simulink model "lqr_design_model"  (R2024a)
settings: Solver=ode45  StartTime=0.0  StopTime=2  FixedStep=0.002  RelTol=1e-3  EnableMultiTasking=on
values from neighbouring files (symbols this model uses):
  A = [0, 0, 1, 0 ... (first row only)    [Torsion_1D_ABCD_eqns_student.m]
  B = Kg * eta_g * kt * eta_m * B / Rm    [Torsion_1D_ABCD_eqns_student.m]
  C = [1, 0, 0, 0 ... (first row only)    [Torsion_1D_ABCD_eqns_student.m]    (also in pid_design.m = pid(Kp, Ki, Kd))
  K = db2mag(12.15)    [pid_design.m]    (also in setup_torsion.m = d_torsion_1d_lqr(A,B))
libraries: quarc_library x2
settings Model: ExtModeTrigDuration=10000  Creator=quarc_user  LastModifiedBy=quarc_user
settings SolverCC: AlgebraicLoopSolver=TrustRegion  PositivePriorityOrder=on
settings DataIOCC: ReturnWorkspaceOutputs=off
settings DebuggingCC: UnconnectedInputMsg=warning  UnconnectedOutputMsg=warning  UnconnectedLineMsg=warning  ArithmeticOperatorsInVariantConditions=warning
settings ModelReferenceCC: EnableRefExpFcnMdlSchedulingChecks=on
settings SFSimCC: SimUseLocalCustomCode=off  CustomCodeUndefinedFunction=UseInterfaceOnly
settings RTWCC: Description=QUARC Win64 Target Using Toolchain  SystemTargetFile=quarc_win64.tlc  TemplateMakefile=quarc_default_tmf  RTWUseLocalCustomCode=off  Toolchain=QUARC win64 | nmake (64-bit Windows)  BuildConfiguration=Faster Runs  GPUComputeCapability=3.5
settings CodeAppCC: StateflowObjectComments=on
settings STFCustomTargetCC: ConcurrentExecutionCompliant=on  SystemTargetFile=quarc_win64.tlc
settings GRTTargetCC: ParMdlRefBuildCompliant=off  CompOptLevelCompliant=off  CombineOutputUpdateFcns=off  MatFileLogging=off  CPPClassGenCompliant=off  GRTInterface=on  ExtMode=on  ExtModeMexFile=quarc_comm
settings ConfigComp: CovMetricSettings=dswe

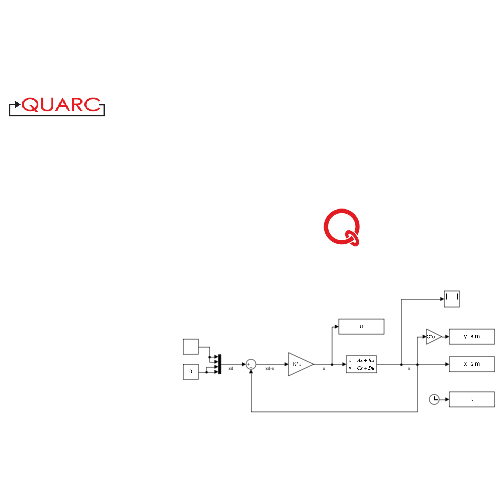
[thumbnail: Simulink's stored preview of the top-level diagram]
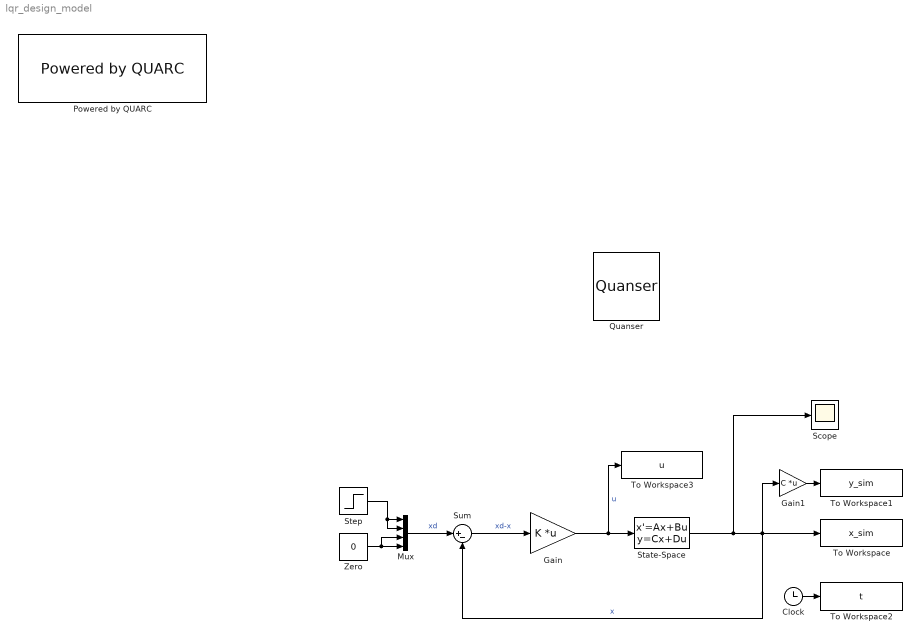
== system lqr_design_model ==
  Clock : Clock
  Gain : Gain  Gain=K  Multiplication=Matrix(K*u)
  Gain1 : Gain  Gain=C  Multiplication=Matrix(K*u)
  Mux : Mux
  Powered by QUARC : quarc_library/Logos/Powered by QUARC
  Quanser : quarc_library/Logos/Quanser
  Scope : Scope
  State-Space : StateSpace  A=A  B=B  C=eye(4)  D=zeros(4,1)  InitialCondition=0
  Step : Step  Time=0  After=10*pi/180  SampleTime=0
  Sum : Sum  Inputs=|+-
  To Workspace : ToWorkspace  VariableName=x_sim  SampleTime=-1
  To Workspace1 : ToWorkspace  VariableName=y_sim  SampleTime=-1
  To Workspace2 : ToWorkspace  VariableName=t  SampleTime=-1
  To Workspace3 : ToWorkspace  VariableName=u  SampleTime=-1
  Zero : Constant  Value=0  OutDataTypeStr=Inherit: Inherit via back propagation
  wires:
  Gain/1 -> To Workspace3/1, State-Space/1  "u"
  Sum/1 -> Gain/1  "xd-x"
  State-Space/1 -> Scope/1, Gain1/1, Sum/2, To Workspace/1  "x"
  Step/1 -> Mux/2, Mux/1
  Mux/1 -> Sum/1  "xd"
  Zero/1 -> Mux/3, Mux/4
  Gain1/1 -> To Workspace1/1
  Clock/1 -> To Workspace2/1
